simulink model "lab_lf"  (R2023a)
settings: Solver=VariableStepAuto  StartTime=0.0  StopTime=inf  RelTol=1e-3
undefined symbols (not defined in the file): National_Instruments, PCI
libraries: sldrtlib x3, slpidlib x1
settings Model: Creator=EAL  LastModifiedBy=EAL

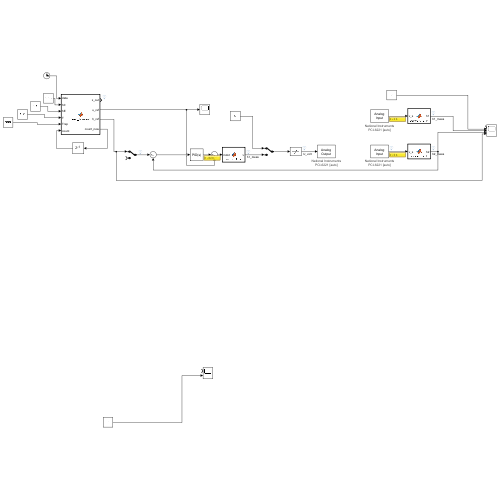
[thumbnail: Simulink's stored preview of the top-level diagram]
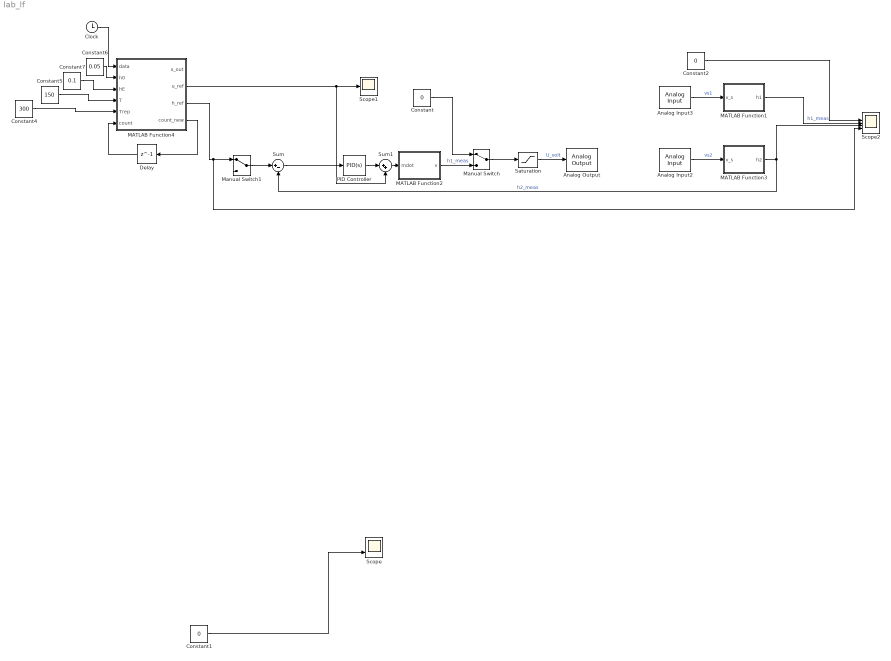
== system lab_lf ==
  Analog Input2 : sldrtlib/Analog Input  SampleTime=0.1  MaxMissedTicks=10  ShowMissedTicks=off  YieldWhenWaiting=off  DrvName=National_Instruments/PCI-6221  DrvAddress=4294967295  DrvOptions=[0 4 0 0 0]  Channels=1  RangeMode=1  VoltRange=1  DataType=1
      settings: AttributesFormatString=National Instruments\nPCI-6221 [auto]
  Analog Input3 : sldrtlib/Analog Input  SampleTime=0.1  MaxMissedTicks=10  ShowMissedTicks=off  YieldWhenWaiting=off  DrvName=National_Instruments/PCI-6221  DrvAddress=4294967295  DrvOptions=[0 4 0 0 0]  Channels=1  RangeMode=1  VoltRange=1  DataType=1
      settings: AttributesFormatString=National Instruments\nPCI-6221 [auto]
  Analog Output : sldrtlib/Analog Output  SampleTime=0.1  MaxMissedTicks=10  ShowMissedTicks=off  YieldWhenWaiting=off  DrvName=National_Instruments/PCI-6221  DrvAddress=4294967295  DrvOptions=[0 4 0 0 0]  Channels=1  RangeMode=1  VoltRange=1  InitialValue=[]  FinalValue=[]
      settings: AttributesFormatString=National Instruments\nPCI-6221 [auto]
  Clock : Clock
  Constant : Constant  Value=0
  Constant1 : Constant  Value=0
  Constant2 : Constant  Value=0
  Constant4 : Constant  Value=300
  Constant5 : Constant  Value=150
  Constant6 : Constant  Value=0.05
  Constant7 : Constant  Value=0.1
  Delay : Delay  DelayLength=1
  MATLAB Function1 : MATLAB Function  TreatAsAtomicUnit=on
  MATLAB Function2 : MATLAB Function  TreatAsAtomicUnit=on
  MATLAB Function3 : MATLAB Function  TreatAsAtomicUnit=on
  MATLAB Function4 : MATLAB Function  TreatAsAtomicUnit=on
  Manual Switch : ManualSwitch
  Manual Switch1 : ManualSwitch
  PID Controller : slpidlib/PID Controller  Controller=PID  Form=Parallel  TimeDomain=Continuous-time  UseExternalTs=off  SampleTime=-1  IntegratorMethod=Forward Euler  FilterMethod=Forward Euler  ControllerParametersSource=internal  P=43  I=3  UseKiTs=off  D=0  N=10  UseFilter=on  TunerSelectOption=Transfer Function Based (PID Tuner App)  InitialConditionSource=internal  InitialConditionForIntegrator=0  InitialConditionForFilter=0  DifferentiatorICPrevScaledInput=0  ExternalReset=none  TrackingMode=off  Kt=1  LimitOutput=off  SatLimitsSource=internal  UpperSaturationLimit=inf  LowerSaturationLimit=-inf  LinearizeAsGain=on  AntiWindupMode=none  Kb=1  LimitIntegrator=off  UpperIntegratorSaturationLimit=inf  LowerIntegratorSaturationLimit=-inf  POutMin=[]  POutMax=[]  IOutMin=[]  IOutMax=[]  DOutMin=[]  DOutMax=[]  NOutMin=[]  NOutMax=[]  SumOutMin=[]  SumOutMax=[]  SaturationOutMin=[]  SaturationOutMax=[]  PParamMin=[]  PParamMax=[]  IParamMin=[]  IParamMax=[]  DParamMin=[]  DParamMax=[]  NParamMin=[]  NParamMax=[]  KbParamMin=[]  KbParamMax=[]  KtParamMin=[]  KtParamMax=[]  KbOutMin=[]  KbOutMax=[]  KtOutMin=[]  KtOutMax=[]  IntegratorOutMin=[]  IntegratorOutMax=[]  FilterOutMin=[]  FilterOutMax=[]  SumI1OutMin=[]  SumI1OutMax=[]  SumI2OutMin=[]  SumI2OutMax=[]  SumI3OutMin=[]  SumI3OutMax=[]  SumI4OutMin=[]  SumI4OutMax=[]  SumDOutMin=[]  SumDOutMax=[]  DifferentiatorOutMin=[]  DifferentiatorOutMax=[]  FilterDiffOutCoefMin=[]  FilterDiffOutCoefMax=[]  ReciprocalOutMin=[]  ReciprocalOutMax=[]  SumDenOutMin=[]  SumDenOutMax=[]  SumNumOutMin=[]  SumNumOutMax=[]  DivideOutMin=[]  DivideOutMax=[]  UdiffTsProdOutMin=[]  UdiffTsProdOutMax=[]  NTsProdOutMin=[]  NTsProdOutMax=[]  UintegralTsProdOutMin=[]  UintegralTsProdOutMax=[]  UngainTsProdOutMin=[]  UngainTsProdOutMax=[]  ClampingZeroOutDataTypeStr=Inherit: Inherit via back propagation  ClampingZeroOutMin=[]  ClampingZeroOutMax=[]  FilterDenConstantOutDataTypeStr=Inherit: Inherit via back propagation  FilterDenConstantOutMin=[]  FilterDenConstantOutMax=[]  PCopyOutDataTypeStr=Inherit: Inherit via back propagation  PCopyOutMin=[]  PCopyOutMax=[]  NCopyOutDataTypeStr=Inherit: Inherit via back propagation  NCopyOutMin=[]  NCopyOutMax=[]  IntegratorContinuousStateAttributes=''  IntegratorStateMustResolveToSignalObject=off  IntegratorRTWStateStorageClass=Auto  FilterContinuousStateAttributes=''  FilterStateMustResolveToSignalObject=off  FilterRTWStateStorageClass=Auto  ParallelPVariant=InternalParameters  IdealPVariant=Disabled  IVariant=InternalParameters  DVariant=InternalParameters  IntegratorVariant=Continuous  SatVariant=Disabled  AWVariant=Passthrough  PCopyVariant=Disabled  TRVariant=Disabled  FdbkBlocksVariant=Forward  IdealPFdbkVariant=Disabled  SatFdbkVariant=Disabled  DerivativeFilterVariant=ContFilter  NVariant=InternalParameters  NCopyVariant=Disabled  FilterICVariant=InternalICsFilter  IntegratorICVariant=InternalICs  ExternalResetVariant=Disabled  TRSumVariant=Passthrough  SumFdbkVariant=Disabled  SumVariant=Sum_PID  TsampFilterVariant=InternalTs  TsampNgainVariant=Passthrough  TsampIntegralVariant=Disabled_SignalSpec  ExternalSaturationOutDataTypeStr=Inherit: Same as second input
  Saturation : Saturate  UpperLimit=5  LowerLimit=0
  Scope : Scope  NumInputPorts=2
  Scope1 : Scope
  Scope2 : Scope  NumInputPorts=5
  Sum : Sum  Inputs=|+-
  Sum1 : Sum  Inputs=|++
  wires:
  Constant1/1 -> Scope/2
  MATLAB Function3/1(h2) -> Scope2/4, Sum/2  "h2_meas"
  Saturation/1 -> Analog Output/1  "U_volt"
  Constant2/1 -> Scope2/2
  MATLAB Function1/1(h1) -> Scope2/3  "h1_meas"
  Manual Switch/1 -> Saturation/1
  Constant/1 -> Manual Switch/1
  MATLAB Function2/1(v) -> Manual Switch/2  "h1_meas"
  Manual Switch1/1 -> Sum/1
  Analog Input2/1 -> MATLAB Function3/1(v_s)  "vs2"
  Analog Input3/1 -> MATLAB Function1/1(v_s)  "vs1"
  PID Controller/1 -> Sum1/1
  Sum1/1 -> MATLAB Function2/1(mdot)
  MATLAB Function4/2(u_ref) -> Scope1/1, Sum1/2
  MATLAB Function4/3(h_ref) -> Scope2/5, Manual Switch1/1
  Constant6/1 -> MATLAB Function4/2(h0)
  Constant7/1 -> MATLAB Function4/3(hE)
  Constant5/1 -> MATLAB Function4/4(T)
  MATLAB Function4/4(count_new) -> Delay/1
  Delay/1 -> MATLAB Function4/6(count)
  Constant4/1 -> MATLAB Function4/5(Trep)
  Sum/1 -> PID Controller/1
  Clock/1 -> MATLAB Function4/1(data)

== matlab function lab_lf/MATLAB Function1 ==
  data: v_s input; h1 output
function h1 = convert_2_h(v_s)
h1 = 0.1347 *v_s -0.2871;

== matlab function lab_lf/MATLAB Function2 ==
  data: mdot input; v output
function v = mdot_2_v(mdot)
k_pump = 0.0167;
v = mdot / k_pump;

== matlab function lab_lf/MATLAB Function4 ==
  data: data input; h0 input; hE input; T input; Trep input; count input; x_out output; u_ref output; h_ref output; count_new output
function [x_out,u_ref,h_ref,count_new] = feed_forward(data, h0,hE,T,Trep,count)
t = data-Trep;
count_new = count+1;
dT = 0.1;
t = count_new*dT;

if mod(floor(t/Trep), 2)
    h0_traj = hE;
    hE_traj = h0;
else
    h0_traj = h0;
    hE_traj = hE;
end
    
a_1 = 0.0574;
a_2 = 0.0524;
rho = 1000;
A_t = 50e-4;

% Calculate Trajectory
x_ref = 0;
xp_ref = 0;
xpp_ref = 0;


tau = rem(t, Trep);

if tau > T
    x_ref = hE_traj;
else
    a0 = h0_traj;
    a1 = 0;
    a2 = 0;
    a3 = 10*(hE_traj-h0_traj)/T^3;
    a4 = -15*(hE_traj-h0_traj)/T^4;
    a5 = 6*(hE_traj-h0_traj)/T^5;
    x_ref = a0 + a3*tau^3 + a4*tau^4 + a5*tau^5;
    xp_ref = 3*a3*tau^2 + 4*a4*tau^3 + 5*a5*tau^4;
    xpp_ref = 6*a3*tau + 12*a4*tau^2 + 20*a5*tau^3;
end

h1 = (xp_ref + a_2*sqrt(x_ref))^2 / a_1^2;
h1_dot = 2/a_1^2 * (xp_ref + a_2*sqrt(x_ref)) * (xpp_ref + a_2*xp_ref/(2*sqrt(x_ref)));
u_ref = rho*A_t * (h1_dot + a_1*sqrt(h1));
h_ref = x_ref; 
x_out = [x_ref,xp_ref,xpp_ref,h1,h1_dot]';
end

== matlab function lab_lf/MATLAB Function3 ==
  data: v_s input; h2 output
function h2 = convert_2_h(v_s)
h2 = 0.1394 *v_s -0.2909;
